simulink model "rocket_withwind"  (R2023a)
settings: Solver=ode15s  StartTime=0.0  StopTime=400  RelTol=1e-3
libraries: vrlib x2, slpidlib x2, shared6dof x1, aerolibadyn x1
settings Model: Creator=kaleb  LastModifiedBy=kaleb

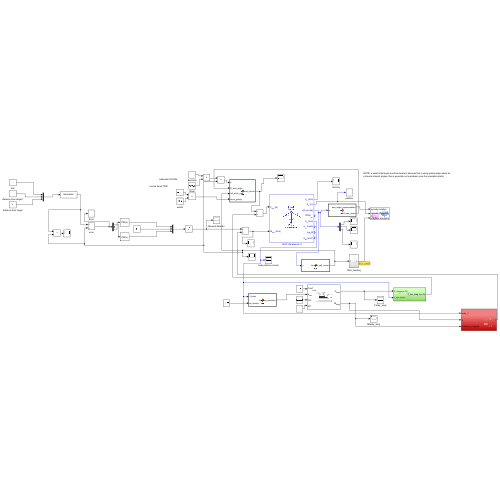
[thumbnail: Simulink's stored preview of the top-level diagram]
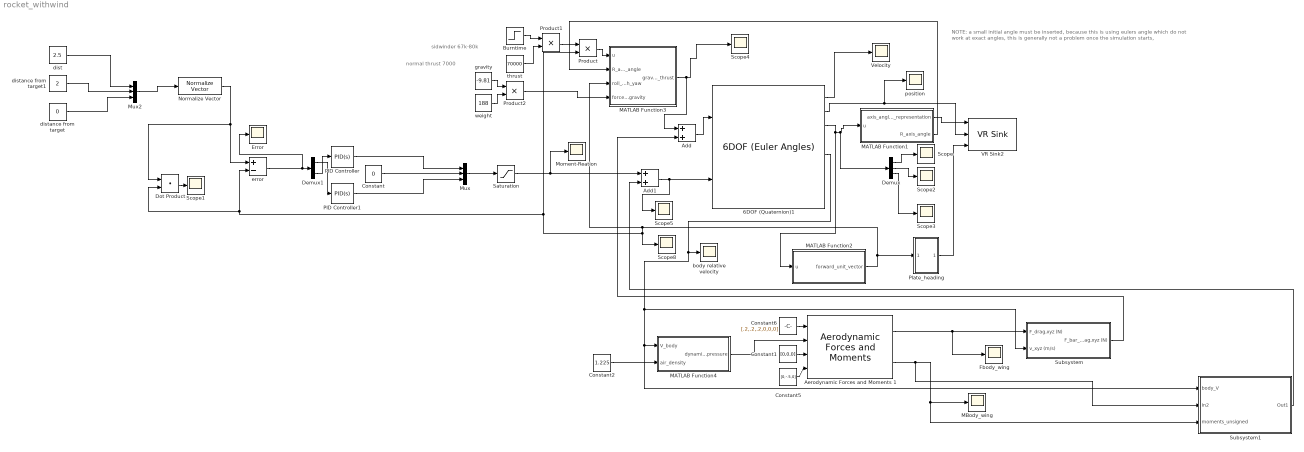
== system rocket_withwind ==
  note: sidwinder 67k-80k
  note: normal thrust 7000
  note: NOTE: a small initial angle must be inserted, because this is using eulers angle which do not work at exact angles, this is generally not a problem once the simulation starts,
  6DOF (Quaternion)1 : shared6dof/6DOF (Euler Angles)  units=Metric (MKS)  mtype=Fixed  rep=Quaternion  xme_0=[0 20 0]  Vm_0=[0 0 0]  eul_0=[0 0 pi/2.5]  pm_0=[0 0 0]  mass_0=188  mass_e=0.5  mass_f=2.0  inertia=[1000,0,0;0,100,0;0,0,1000]  inertia_e=eye(3)  inertia_f=2*eye(3)  k_quat=1  vre_flag=on  abi_flag=off  aMode=0  xme_statename=''  Vm_statename=''  eul_statename=''  quat_statename=''  pm_statename=''  mass_statename=''
  Add : Sum
  Add1 : Sum
  Aerodynamic Forces and Moments 1 : aerolibadyn/Aerodynamic Forces and Moments   inputAxes=Body  outputForceAxes=Body  outputMomentAxes=Body  S=1  b=1  cbar=1
  Burntime : Step  Time=30  Before=1  After=0  SampleTime=0
  Constant : Constant  Value=0
  Constant1 : Constant  Value=[0,0,0]
  Constant2 : Constant  Value=1.225
  Constant5 : Constant  Value=[0,-.5,0]
  Constant6 : Constant  Value=[.2,.2,.2,0,0,0]
  Demux : Demux  Outputs=3
  Demux1 : Demux  Outputs=3
  Dot Product : DotProduct  OutDataTypeStr=Inherit: Inherit via internal rule
  Error : Scope
  Fbody_wing : Scope
  MATLAB Function1 : MATLAB Function  TreatAsAtomicUnit=on
  MATLAB Function2 : MATLAB Function  TreatAsAtomicUnit=on
  MATLAB Function3 : MATLAB Function  TreatAsAtomicUnit=on
  MATLAB Function4 : MATLAB Function  TreatAsAtomicUnit=on
  MBody_wing : Scope
  Moment-Reation : Scope
  Mux : Mux  Inputs=3
  Mux2 : Mux  Inputs=3
  Normalize Vector : vrlib/Utilities/Normalize Vector  maxzero=0
  PID Controller : slpidlib/PID Controller  Controller=PID  Form=Parallel  TimeDomain=Continuous-time  UseExternalTs=off  SampleTime=-1  IntegratorMethod=Forward Euler  FilterMethod=Forward Euler  ControllerParametersSource=internal  P=65.9286050437834  I=0.609586047559938  UseKiTs=off  D=1584.28651897464  N=181.126027938245  UseFilter=on  TunerSelectOption=Transfer Function Based (PID Tuner App)  InitialConditionSource=internal  InitialConditionForIntegrator=0  InitialConditionForFilter=0  DifferentiatorICPrevScaledInput=0  ExternalReset=none  TrackingMode=off  Kt=1  LimitOutput=off  SatLimitsSource=internal  UpperSaturationLimit=inf  LowerSaturationLimit=-inf  LinearizeAsGain=on  AntiWindupMode=none  Kb=1  LimitIntegrator=off  UpperIntegratorSaturationLimit=inf  LowerIntegratorSaturationLimit=-inf  POutMin=[]  POutMax=[]  IOutMin=[]  IOutMax=[]  DOutMin=[]  DOutMax=[]  NOutMin=[]  NOutMax=[]  SumOutMin=[]  SumOutMax=[]  SaturationOutMin=[]  SaturationOutMax=[]  PParamMin=[]  PParamMax=[]  IParamMin=[]  IParamMax=[]  DParamMin=[]  DParamMax=[]  NParamMin=[]  NParamMax=[]  KbParamMin=[]  KbParamMax=[]  KtParamMin=[]  KtParamMax=[]  KbOutMin=[]  KbOutMax=[]  KtOutMin=[]  KtOutMax=[]  IntegratorOutMin=[]  IntegratorOutMax=[]  FilterOutMin=[]  FilterOutMax=[]  SumI1OutMin=[]  SumI1OutMax=[]  SumI2OutMin=[]  SumI2OutMax=[]  SumI3OutMin=[]  SumI3OutMax=[]  SumI4OutMin=[]  SumI4OutMax=[]  SumDOutMin=[]  SumDOutMax=[]  DifferentiatorOutMin=[]  DifferentiatorOutMax=[]  FilterDiffOutCoefMin=[]  FilterDiffOutCoefMax=[]  ReciprocalOutMin=[]  ReciprocalOutMax=[]  SumDenOutMin=[]  SumDenOutMax=[]  SumNumOutMin=[]  SumNumOutMax=[]  DivideOutMin=[]  DivideOutMax=[]  UdiffTsProdOutMin=[]  UdiffTsProdOutMax=[]  NTsProdOutMin=[]  NTsProdOutMax=[]  UintegralTsProdOutMin=[]  UintegralTsProdOutMax=[]  UngainTsProdOutMin=[]  UngainTsProdOutMax=[]  ClampingZeroOutDataTypeStr=Inherit: Inherit via back propagation  ClampingZeroOutMin=[]  ClampingZeroOutMax=[]  FilterDenConstantOutDataTypeStr=Inherit: Inherit via back propagation  FilterDenConstantOutMin=[]  FilterDenConstantOutMax=[]  PCopyOutDataTypeStr=Inherit: Inherit via back propagation  PCopyOutMin=[]  PCopyOutMax=[]  NCopyOutDataTypeStr=Inherit: Inherit via back propagation  NCopyOutMin=[]  NCopyOutMax=[]  IntegratorContinuousStateAttributes=''  IntegratorStateMustResolveToSignalObject=off  IntegratorRTWStateStorageClass=Auto  FilterContinuousStateAttributes=''  FilterStateMustResolveToSignalObject=off  FilterRTWStateStorageClass=Auto  ParallelPVariant=InternalParameters  IdealPVariant=Disabled  IVariant=InternalParameters  DVariant=InternalParameters  IntegratorVariant=Continuous  SatVariant=Disabled  AWVariant=Passthrough  PCopyVariant=Disabled  TRVariant=Disabled  FdbkBlocksVariant=Forward  IdealPFdbkVariant=Disabled  SatFdbkVariant=Disabled  DerivativeFilterVariant=ContFilter  NVariant=InternalParameters  NCopyVariant=Disabled  FilterICVariant=InternalICsFilter  IntegratorICVariant=InternalICs  ExternalResetVariant=Disabled  TRSumVariant=Passthrough  SumFdbkVariant=Disabled  SumVariant=Sum_PID  TsampFilterVariant=InternalTs  TsampNgainVariant=Passthrough  TsampIntegralVariant=Disabled_SignalSpec  ExternalSaturationOutDataTypeStr=Inherit: Same as second input
  PID Controller1 : slpidlib/PID Controller  Controller=PID  Form=Parallel  TimeDomain=Continuous-time  UseExternalTs=off  SampleTime=-1  IntegratorMethod=Forward Euler  FilterMethod=Forward Euler  ControllerParametersSource=internal  P=-2624.66504124445  I=-153.121092169898  UseKiTs=off  D=-9996.1721490515  N=1142.8279760416  UseFilter=on  TunerSelectOption=Transfer Function Based (PID Tuner App)  InitialConditionSource=internal  InitialConditionForIntegrator=0  InitialConditionForFilter=0  DifferentiatorICPrevScaledInput=0  ExternalReset=none  TrackingMode=off  Kt=1  LimitOutput=off  SatLimitsSource=internal  UpperSaturationLimit=inf  LowerSaturationLimit=-inf  LinearizeAsGain=on  AntiWindupMode=none  Kb=1  LimitIntegrator=off  UpperIntegratorSaturationLimit=inf  LowerIntegratorSaturationLimit=-inf  POutMin=[]  POutMax=[]  IOutMin=[]  IOutMax=[]  DOutMin=[]  DOutMax=[]  NOutMin=[]  NOutMax=[]  SumOutMin=[]  SumOutMax=[]  SaturationOutMin=[]  SaturationOutMax=[]  PParamMin=[]  PParamMax=[]  IParamMin=[]  IParamMax=[]  DParamMin=[]  DParamMax=[]  NParamMin=[]  NParamMax=[]  KbParamMin=[]  KbParamMax=[]  KtParamMin=[]  KtParamMax=[]  KbOutMin=[]  KbOutMax=[]  KtOutMin=[]  KtOutMax=[]  IntegratorOutMin=[]  IntegratorOutMax=[]  FilterOutMin=[]  FilterOutMax=[]  SumI1OutMin=[]  SumI1OutMax=[]  SumI2OutMin=[]  SumI2OutMax=[]  SumI3OutMin=[]  SumI3OutMax=[]  SumI4OutMin=[]  SumI4OutMax=[]  SumDOutMin=[]  SumDOutMax=[]  DifferentiatorOutMin=[]  DifferentiatorOutMax=[]  FilterDiffOutCoefMin=[]  FilterDiffOutCoefMax=[]  ReciprocalOutMin=[]  ReciprocalOutMax=[]  SumDenOutMin=[]  SumDenOutMax=[]  SumNumOutMin=[]  SumNumOutMax=[]  DivideOutMin=[]  DivideOutMax=[]  UdiffTsProdOutMin=[]  UdiffTsProdOutMax=[]  NTsProdOutMin=[]  NTsProdOutMax=[]  UintegralTsProdOutMin=[]  UintegralTsProdOutMax=[]  UngainTsProdOutMin=[]  UngainTsProdOutMax=[]  ClampingZeroOutDataTypeStr=Inherit: Inherit via back propagation  ClampingZeroOutMin=[]  ClampingZeroOutMax=[]  FilterDenConstantOutDataTypeStr=Inherit: Inherit via back propagation  FilterDenConstantOutMin=[]  FilterDenConstantOutMax=[]  PCopyOutDataTypeStr=Inherit: Inherit via back propagation  PCopyOutMin=[]  PCopyOutMax=[]  NCopyOutDataTypeStr=Inherit: Inherit via back propagation  NCopyOutMin=[]  NCopyOutMax=[]  IntegratorContinuousStateAttributes=''  IntegratorStateMustResolveToSignalObject=off  IntegratorRTWStateStorageClass=Auto  FilterContinuousStateAttributes=''  FilterStateMustResolveToSignalObject=off  FilterRTWStateStorageClass=Auto  ParallelPVariant=InternalParameters  IdealPVariant=Disabled  IVariant=InternalParameters  DVariant=InternalParameters  IntegratorVariant=Continuous  SatVariant=Disabled  AWVariant=Passthrough  PCopyVariant=Disabled  TRVariant=Disabled  FdbkBlocksVariant=Forward  IdealPFdbkVariant=Disabled  SatFdbkVariant=Disabled  DerivativeFilterVariant=ContFilter  NVariant=InternalParameters  NCopyVariant=Disabled  FilterICVariant=InternalICsFilter  IntegratorICVariant=InternalICs  ExternalResetVariant=Disabled  TRSumVariant=Passthrough  SumFdbkVariant=Disabled  SumVariant=Sum_PID  TsampFilterVariant=InternalTs  TsampNgainVariant=Passthrough  TsampIntegralVariant=Disabled_SignalSpec  ExternalSaturationOutDataTypeStr=Inherit: Same as second input
  Plate_heading : Subsystem
  Product : Product
  Product1 : Product
  Product2 : Product
  Saturation : Saturate  UpperLimit=2000  LowerLimit=-2000
  Scope{,1..5,8} (7 alike) : Scope
  Subsystem : Subsystem
  Subsystem1 : Subsystem
  VR Sink2 : vrlib/VR Sink  InstantiateOnLoad=on  SampleTime=0.1  ViewEnable=on  RemoteChange=off  RemoteView=off  FieldsWritten=cylinder.rotation.4.1.1.double#cylinder.translation.3.1.1.double#my_floor.translation.3.1.1.double  WorldFileName=C:\Users\kaleb\Downloads\cylinderfallbackground.wrl  AutoView=off  VideoDimensions=[]  AllowVariableSize=off
  Velocity : Scope
  body relative velocity : Scope
  dist : Constant  Value=2.5
  distance from target : Constant  Value=0
  distance from target1 : Constant  Value=2
  error : Sum  Inputs=+-
  gravity : Constant  Value=-9.81
  position : Scope
  thrust : Constant  Value=70000
  weight : Constant  Value=188
  wires:
  Saturation/1 -> Add1/1, Moment-Reation/1
  MATLAB Function1/2(R_axis_angle) -> MATLAB Function3/2(R_axis_angle)
  PID Controller1/1 -> Mux/3
  Mux/1 -> Saturation/1
  PID Controller/1 -> Mux/1
  Demux1/1 -> PID Controller1/1
  MATLAB Function2/1(forward_unit_vector) -> MATLAB Function3/3(roll_pitch_yaw), Scope8/1, Product/2, Dot Product/2, error/2, Plate_heading/1(In1)
  Burntime/1 -> Product1/1
  MATLAB Function1/1(axis_angle_representation) -> VR Sink2/1
  6DOF (Quaternion)1/1 -> Velocity/1
  Product1/1 -> Product/1
  Demux/1 -> Scope/1
  gravity/1 -> Product2/1
  Product2/1 -> MATLAB Function3/4(force_gravity)
  MATLAB Function3/1(gravity_thrust) -> Add/1, Scope4/1
  Demux/3 -> Scope3/1
  6DOF (Quaternion)1/3 -> MATLAB Function2/1(u), Demux/1, MATLAB Function1/1(u)
  thrust/1 -> Product1/2
  Demux/2 -> Scope2/1
  Constant/1 -> Mux/2
  Normalize Vector/1 -> Dot Product/1, error/1
  weight/1 -> Product2/2
  Product/1 -> MATLAB Function3/1(u)
  Demux1/3 -> PID Controller/1
  error/1 -> Error/1, Demux1/1
  Dot Product/1 -> Scope1/1
  dist/1 -> Mux2/1
  distance from target1/1 -> Mux2/2
  distance from target/1 -> Mux2/3
  Mux2/1 -> Normalize Vector/1
  6DOF (Quaternion)1/5 -> Subsystem/2(v_xyz (m/s)), Subsystem1/1(body_V), MATLAB Function4/1(V_body), body relative velocity/1
  Constant1/1 -> Aerodynamic Forces and Moments 1/3
  Constant5/1 -> Aerodynamic Forces and Moments 1/4
  Constant6/1 -> Aerodynamic Forces and Moments 1/1
  Aerodynamic Forces and Moments 1/2 -> Subsystem1/2(In2), Subsystem1/3(moments_unsigned), MBody_wing/1
  Constant2/1 -> MATLAB Function4/2(air_density)
  MATLAB Function4/1(dynamic_pressure) -> Aerodynamic Forces and Moments 1/2
  Aerodynamic Forces and Moments 1/1 -> Subsystem/1(F_drag,xyz (N)), Fbody_wing/1
  6DOF (Quaternion)1/2 -> position/1, VR Sink2/2
  Add/1 -> 6DOF (Quaternion)1/1
  Subsystem/1(F_bar_drag,xyz (N)) -> Add/2
  Add1/1 -> 6DOF (Quaternion)1/2, Scope5/1
  Subsystem1/1(Out1) -> Add1/2
  Plate_heading/1(Out1) -> VR Sink2/3

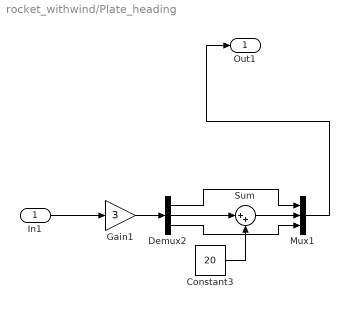
== system rocket_withwind/Plate_heading ==
  In1 : Inport
  Constant3 : Constant  Value=20
  Demux2 : Demux  Outputs=3
  Gain1 : Gain  Gain=3
  Mux1 : Mux  Inputs=3
  Sum : Sum  Inputs=|++
  Out1 : Outport
  wires:
  Mux1/1 -> Out1/1
  Constant3/1 -> Sum/2
  Demux2/1 -> Mux1/1
  Gain1/1 -> Demux2/1
  Demux2/2 -> Sum/1
  Sum/1 -> Mux1/2
  In1/1 -> Gain1/1
  Demux2/3 -> Mux1/3

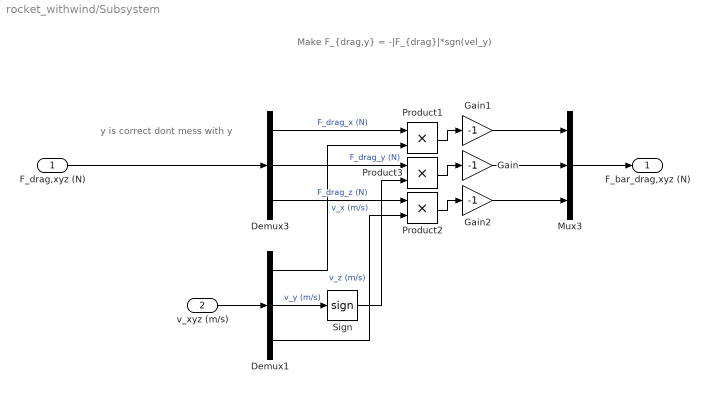
== system rocket_withwind/Subsystem ==
  note: y is correct dont mess with y
  note: Make F_{drag,y} = -|F_{drag}|*sgn(vel_y)
  F_drag,xyz (N) : Inport
  v_xyz (m/s) : Inport  Port=2
  Demux1 : Demux  Outputs=3
  Demux3 : Demux  Outputs=3
  Gain : Gain  Gain=-1
  Gain1 : Gain  Gain=-1
  Gain2 : Gain  Gain=-1
  Mux3 : Mux  Inputs=3
  Product1 : Product
  Product2 : Product
  Product3 : Product
  Sign : Signum
  F_bar_drag,xyz (N) : Outport
  wires:
  Demux1/2 -> Sign/1  "v_y (m/s)"
  v_xyz (m/s)/1 -> Demux1/1
  Demux1/1 -> Product1/2  "v_x (m/s)"
  Demux1/3 -> Product2/2  "v_z (m/s)"
  Gain/1 -> Mux3/2
  Mux3/1 -> F_bar_drag,xyz (N)/1
  F_drag,xyz (N)/1 -> Demux3/1
  Demux3/2 -> Product3/1  "F_drag_y (N)"
  Product3/1 -> Gain/1
  Sign/1 -> Product3/2
  Product1/1 -> Gain1/1
  Demux3/1 -> Product1/1  "F_drag_x (N)"
  Gain1/1 -> Mux3/1
  Product2/1 -> Gain2/1
  Demux3/3 -> Product2/1  "F_drag_z (N)"
  Gain2/1 -> Mux3/3

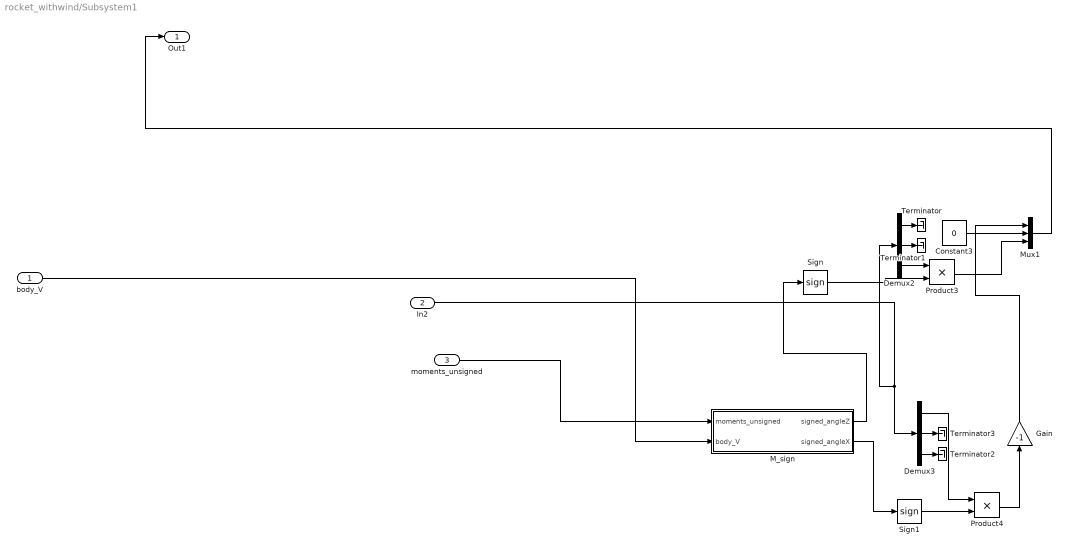
== system rocket_withwind/Subsystem1 ==
  body_V : Inport
  In2 : Inport  Port=2
  moments_unsigned : Inport  Port=3
  Constant3 : Constant  Value=0
  Demux2 : Demux  Outputs=3
  Demux3 : Demux  Outputs=3
  Gain : Gain  Gain=-1
  M_sign : MATLAB Function  TreatAsAtomicUnit=on
  Mux1 : Mux  Inputs=3
  Product3 : Product
  Product4 : Product
  Sign : Signum
  Sign1 : Signum
  Terminator{,1..3} (4 alike) : Terminator
  Out1 : Outport
  wires:
  Sign/1 -> Product3/2
  Product3/1 -> Mux1/3
  body_V/1 -> M_sign/2(body_V)
  Demux3/1 -> Product4/1
  In2/1 -> Demux3/1, Demux2/1
  M_sign/1(signed_angleZ) -> Sign/1
  Product4/1 -> Gain/1
  Demux2/3 -> Product3/1
  Constant3/1 -> Mux1/2
  M_sign/2(signed_angleX) -> Sign1/1
  Sign1/1 -> Product4/2
  Gain/1 -> Mux1/1
  Demux2/2 -> Terminator1/1
  moments_unsigned/1 -> M_sign/1(moments_unsigned)
  Demux2/1 -> Terminator/1
  Demux3/3 -> Terminator2/1
  Demux3/2 -> Terminator3/1
  Mux1/1 -> Out1/1

== matlab function rocket_withwind/MATLAB Function1 ==
  data: u input; axis_angle_representation output; R_axis_angle output
function [axis_angle_representation, R_axis_angle] = fcn(u)

%this converts euler anlges to axis-angle representation,
%this is needed because Vsink uses that format
roll = u(1);
pitch = u(2);
yaw = u(3);

% Calculate rotation matrix
Rz = [cos(yaw), -sin(yaw), 0;
      sin(yaw), cos(yaw), 0;
      0, 0, 1];
Ry = [cos(pitch), 0, sin(pitch);
      0, 1, 0;
      -sin(pitch), 0, cos(pitch)];
Rx = [1, 0, 0;
      0, cos(roll), -sin(roll);
      0, sin(roll), cos(roll)];

R = Rz * Ry * Rx; % Apply in ZYX order

% Calculate axis and angle from rotation matrix
angle = acos((trace(R) - 1) / 2); % Angle in radians

axis = (1 / (2 * sin(angle))) * [R(3,2) - R(2,3); R(1,3) - R(3,1); R(2,1) - R(1,2)];



%THIS IS A WAY TO AVOID A DIVIDE BY ZERO ERROR, QUATERIONS WOULD BE BETTER
%BUT I THINK THIS ALSO WORKS, but this also makes the code veiw a heading
%directly up and down as the same thing
%disp(axis)
%hasnan = sum(isnan(axis(:)))
%disp(hasnan)
normalized_axis = axis / norm(axis);

if sum(isnan(axis(:))) > 0
    %disp('almost zero')

    %DOUBLE CHECK THIS AXIS I HAVE DOUBTS
    %HHHHHHHHHHHHHHHHHHHHHHHHHHHHHHHHHHHHHHHHHHHHHHHHHHHHHHHH
    axis = [0;0;0];
    normalized_axis = axis;
end

% Create axis-angle representation
axis_angle_representation = [axis; angle];

%testing below

% Calculate trigonometric components
cos_angle = cos(angle);
sin_angle = sin(angle);
one_minus_cos_angle = 1 - cos_angle;

% Construct the rotation matrix using axis-angle representation
R_axis_angle = [
    cos_angle + normalized_axis(1)^2 * one_minus_cos_angle, ...
    normalized_axis(1) * normalized_axis(2) * one_minus_cos_angle - normalized_axis(3) * sin_angle, ...
    normalized_axis(1) * normalized_axis(3) * one_minus_cos_angle + normalized_axis(2) * sin_angle;
    
    normalized_axis(2) * normalized_axis(1) * one_minus_cos_angle + normalized_axis(3) * sin_angle, ...
    cos_angle + normalized_axis(2)^2 * one_minus_cos_angle, ...
    normalized_axis(2) * normalized_axis(3) * one_minus_cos_angle - normalized_axis(1) * sin_angle;
    
    normalized_axis(3) * normalized_axis(1) * one_minus_cos_angle - normalized_axis(2) * sin_angle, ...
    normalized_axis(3) * normalized_axis(2) * one_minus_cos_angle + normalized_axis(1) * sin_angle, ...
    cos_angle + normalized_axis(3)^2 * one_minus_cos_angle
];


%%%%%%%%%%%%%%%%%%%%%%%%%%%%%%%%%%%%%%%%
%below has stuff that require the robotics toolbox
%provided by gtp
% Calculate rotation matrix
%R = eul2rotm([yaw, pitch, roll], 'ZYX'); % Change the order if needed

% Convert rotation matrix to axis-angle representation
%[rotation_axis, angle] = rotm2axang(R);

% Create axis-angle representation
%axis_angle_representation = [rotation_axis'; angle];

== matlab function rocket_withwind/MATLAB Function2 ==
  data: u input; forward_unit_vector output
function forward_unit_vector = fcn(u)

%this converts euler anlges to axis-angle representation,
%this is needed because Vsink uses that format
roll = u(1);
pitch = u(2);
yaw = u(3);

% Calculate rotation matrix
Rz = [cos(yaw), -sin(yaw), 0;
      sin(yaw), cos(yaw), 0;
      0, 0, 1];
Ry = [cos(pitch), 0, sin(pitch);
      0, 1, 0;
      -sin(pitch), 0, cos(pitch)];
Rx = [1, 0, 0;
      0, cos(roll), -sin(roll);
      0, sin(roll), cos(roll)];

% Calculate rotation matrix
R = [cos(yaw)*cos(pitch), cos(yaw)*sin(pitch)*sin(roll) - sin(yaw)*cos(roll), cos(yaw)*sin(pitch)*cos(roll) + sin(yaw)*sin(roll);
     sin(yaw)*cos(pitch), sin(yaw)*sin(pitch)*sin(roll) + cos(yaw)*cos(roll), sin(yaw)*sin(pitch)*cos(roll) - cos(yaw)*sin(roll);
     -sin(pitch), cos(pitch)*sin(roll), cos(pitch)*cos(roll)];

% Calculate forward unit vector
forward_unit_vector = R(:, 2);

== matlab function rocket_withwind/MATLAB Function3 ==
  data: u input; R_axis_angle input; roll_pitch_yaw input; gravity_thrust output; force_gravity input
function gravity_thrust = fcn(u,R_axis_angle, roll_pitch_yaw, force_gravity)
%this adds gravity to the thrust so that gravity only acts down
world_gravity_force = [0,force_gravity,0]';



%fprintf('R axis angle: \n')
%disp(R_axis_angle)

% Transform the gravity vector to the body's local reference frame
gravity_local = R_axis_angle' * world_gravity_force;

%disp(gravity_local)



gravity_thrust = gravity_local + u;
%fprintf(' %f %f %f ', gravity_thrust(1), gravity_thrust(2), gravity_thrust(3))

%disp(gravity_thrust(1))

%disp(gravity_thrust(2))
%disp(gravity_thrust(3))

== matlab function rocket_withwind/MATLAB Function4 ==
  data: V_body input; dynamic_pressure output; air_density input
function dynamic_pressure = fcn(V_body,air_density)
    dynamic_pressure = .5*air_density*(V_body.^2);

== matlab function rocket_withwind/Subsystem1/M_sign ==
  data: moments_unsigned input; body_V input; signed_angleZ output; signed_angleX output
function [signed_angleZ,signed_angleX]  = fcn( moments_unsigned,body_V)

%dot = x1*x2 + y1*y2       Dot product between [x1, y1] and [x2, y2]
%det = x1*y2 - y1*x2      # Determinant
%angle = atan2(det, dot)  # atan2(y, x) or atan2(sin, cos)


%determine the sign of the moment about the Z-axis
XY_velocity = [body_V(1), body_V(2)];
Y_axis = [0,1];
XY_dot = dot(XY_velocity,Y_axis);
XY_det = XY_velocity(1)*Y_axis(2) - XY_velocity(2)*Y_axis(1);
signed_angleZ = atan2(XY_det,XY_dot);
fprintf('the angleZ is %f',signed_angleZ)

%determine the sign of the moment about the X-axis
YZ_velocity = [body_V(2), body_V(3)];
Z_axis = [1,0];
YZ_dot = dot(YZ_velocity,Z_axis);
YZ_det = YZ_velocity(1)*Z_axis(2) - YZ_velocity(2)*Z_axis(1);
signed_angleX = atan2(YZ_det,YZ_dot);
fprintf('the angleX is %f',signed_angleX)
